simulink model "sampleModel1596_5"  (R2023a)
settings: Solver=VariableStepAuto  StartTime=0.0  StopTime=10.0  RelTol=1e-3
libraries: simulink x2, hdlsllib x2
settings Model: Creator=user1  LastModifiedBy=user1

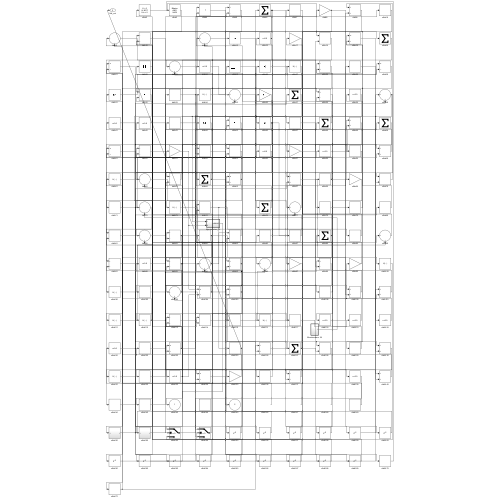
[thumbnail: Simulink's stored preview of the top-level diagram]
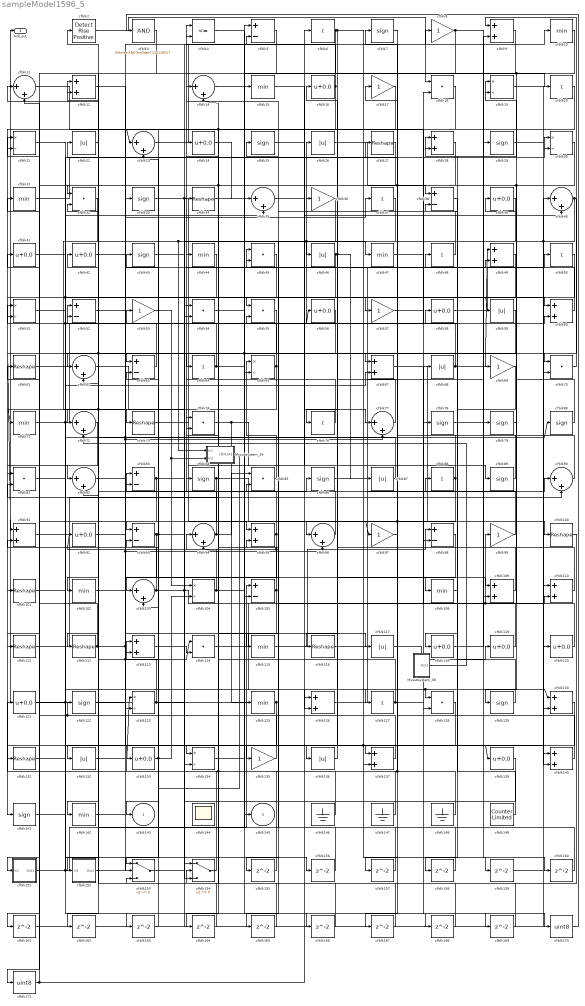
== system sampleModel1596_5 ==
  Mysubsystem_24 : Subsystem  TreatAsAtomicUnit=on  RTWFcnName=Mysubsystem_24
      settings: RTWFcnNameOpts=User specified  RTWFileNameOpts=Use function name
  Mysubsystem_38 : Subsystem  TreatAsAtomicUnit=on  RTWFcnName=Mysubsystem_38
      settings: RTWFcnNameOpts=User specified  RTWFileNameOpts=Use function name
  cfblk{10,15,31,44,47,71,102,108,115,125,142} (11 alike) : MinMax  OutDataTypeStr=uint8
  cfblk{27,34,61,73,100..101,111..112,116,131} (10 alike) : Reshape
  cfblk{11,14,23,35,40,62,72,77,82,90,94,96,103} (13 alike) : Sum  Inputs=|++  OutDataTypeStr=uint8
  cfblk{19,21,30,51,65,104,123,134} (8 alike) : Product  Inputs=*/  OutDataTypeStr=uint8  RndMeth=Zero  SaturateOnIntegerOverflow=on
  cfblk{5,38,52,63,83,93,98,105} (8 alike) : Sum  Inputs=+-  OutDataTypeStr=uint8
  cfblk{9,12,28,49,60,67,91,95,109..110,113,126,130,137,140} (15 alike) : Sum  OutDataTypeStr=uint8
  cfblk{18,32,45,54..55,70,74,81,85,114,128} (11 alike) : DotProduct  OutDataTypeStr=uint8
  cfblk{22,26,46,59,68,87,117,132,136} (9 alike) : Abs  OutDataTypeStr=uint8  SaturateOnIntegerOverflow=off
  cfblk{16,24,39,41..42,56,58,92,118..121,133,139} (14 alike) : Bias  Bias=0.0  SaturateOnIntegerOverflow=off
  cfblk{7,25,29,33,43,78..80,84,86,89,122,129,141} (14 alike) : Signum
  cfblk{6,20,37,48,50,64,76,88,127} (9 alike) : Sum  Inputs=+  OutDataTypeStr=uint8
  cfblk{8,17,36,53,57,69,97,99,135} (9 alike) : Gain  OutDataTypeStr=uint8
  cfblk144 : Scope
      settings: Floating=on
  cfblk146 : Ground
  cfblk147 : Ground
  cfblk148 : Ground
  cfblk149 : hdlsllib/Sources/Counter Limited  uplimit=7  tsamp=-1
  cfblk151 : Subsystem
      settings: LibrarySourceBlock=|
      | hdlsllib/Ports &
      | Subsystems/Subsystem
  cfblk152 : Subsystem
      settings: LibrarySourceBlock=|
      | hdlsllib/Ports &
      | Subsystems/Subsystem
  cfblk153 : Switch  OutDataTypeStr=uint8  SaturateOnIntegerOverflow=off  InputSameDT=off
  cfblk154 : Switch  OutDataTypeStr=uint8  SaturateOnIntegerOverflow=off  InputSameDT=off
  cfblk{155..169} (15 alike) : Delay  SampleTime=1
  cfblk170 : DataTypeConversion  OutDataTypeStr=uint8  SaturateOnIntegerOverflow=off  RndMeth=Floor
  cfblk171 : DataTypeConversion  OutDataTypeStr=uint8  SaturateOnIntegerOverflow=off  RndMeth=Floor
  cfblk2 : hdlsllib/Logic and Bit Operations/Detect Rise Positive  vinit=0  OutDataTypeStr=uint8
  cfblk3 : simulink/Logic and Bit Operations/Bitwise Operator  logicop=AND  UseBitMask=on  BitMask=bin2dec('11011001')  BitMaskRealWorld=Stored Integer
      settings: LibrarySourceBlock=|
      | hdlsllib/Logic and Bit
      | Operations/Bitwise
      | Operator
  cfblk4 : RelationalOperator  Operator=<=  OutDataTypeStr=boolean  InputSameDT=off
  cfblk143 : Outport  OutDataTypeStr=uint8  VectorParamsAs1DForOutWhenUnconnected=off
  cfblk145 : Outport  Port=2  OutDataTypeStr=uint8  VectorParamsAs1DForOutWhenUnconnected=off
  Hdl_out : Outport  Port=3  OutDataTypeStr=uint8
  wires:
  cfblk115/1 -> cfblk98/1
  cfblk53/1 -> cfblk104/1, Mysubsystem_24/2(In2)
  cfblk95/1 -> cfblk4/1, cfblk103/2
  cfblk65/1 -> cfblk71/1, cfblk162/1, cfblk24/1
  cfblk2/1 -> cfblk18/1
  cfblk126/1 -> cfblk48/1
  cfblk6/1 -> cfblk96/1, cfblk159/1, cfblk32/1
  cfblk148/1 -> cfblk123/1, cfblk17/1
  cfblk23/1 -> cfblk10/1
  cfblk110/1 -> cfblk52/1
  cfblk38/1 -> cfblk118/1
  cfblk45/1 -> cfblk133/1
  cfblk68/1 -> cfblk49/1, cfblk51/2
  cfblk33/1 -> cfblk139/1, cfblk137/2, cfblk95/1
  cfblk132/1 -> cfblk114/1, cfblk37/1
  cfblk137/1 -> cfblk113/1
  cfblk32/1 -> cfblk73/1
  cfblk5/1 -> cfblk142/1
  cfblk72/1 -> cfblk141/1
  cfblk74/1 -> cfblk127/1, cfblk125/1
  cfblk113/1 -> cfblk114/2
  cfblk24/1 -> cfblk35/1
  cfblk117/1 -> cfblk119/1
  cfblk76/1 -> cfblk34/1
  cfblk85/1 -> cfblk65/1
  cfblk90/1 -> cfblk22/1
  cfblk93/1 -> cfblk63/2, cfblk85/2, cfblk123/2
  cfblk135/1 -> cfblk122/1, cfblk41/1
  cfblk47/1 -> cfblk98/2
  cfblk26/1 -> cfblk38/1
  cfblk96/1 -> cfblk11/1
  cfblk88/1 -> cfblk44/1, cfblk112/1
  cfblk62/1 -> cfblk154/1
  cfblk18/1 -> cfblk93/1
  cfblk94/1 -> cfblk43/1, cfblk85/1
  cfblk151/1(Out1) -> cfblk105/1, cfblk67/2
  cfblk60/1 -> cfblk25/1
  cfblk71/1 -> cfblk26/1, cfblk140/2
  cfblk43/1 -> cfblk47/1
  cfblk83/1 -> cfblk49/2, cfblk161/1
  cfblk9/1 -> cfblk67/1
  cfblk92/1 -> cfblk8/1, cfblk77/2
  cfblk63/1 -> cfblk11/2
  cfblk127/1 -> cfblk84/1, cfblk169/1
  cfblk89/1 -> cfblk53/1
  cfblk10/1 -> cfblk28/1, cfblk167/1
  cfblk27/1 -> cfblk72/1
  cfblk77/1 -> cfblk16/1
  cfblk21/1 -> cfblk128/1, cfblk130/1, cfblk59/1
  cfblk44/1 -> cfblk153/1
  cfblk52/1 -> cfblk64/1
  cfblk73/1 -> cfblk128/2
  cfblk25/1 -> cfblk40/2
  cfblk67/1 -> cfblk100/1
  cfblk39/1 -> Mysubsystem_24/1(In1), cfblk62/2
  cfblk79/1 -> cfblk19/1
  cfblk133/1 -> cfblk83/1, cfblk104/2
  cfblk114/1 -> cfblk68/1
  cfblk3/1 -> cfblk171/1
  cfblk11/1 -> cfblk78/1
  cfblk123/1 -> cfblk12/1, cfblk60/2
  cfblk48/1 -> cfblk14/1
  cfblk149/1 -> cfblk28/2
  cfblk99/1 -> cfblk42/1
  cfblk70/1 -> cfblk9/1
  cfblk41/1 -> cfblk65/2, cfblk70/2
  cfblk128/1 -> cfblk151/1(In1)
  cfblk147/1 -> cfblk14/2, cfblk61/1
  cfblk116/1 -> cfblk90/1
  cfblk15/1 -> cfblk89/1
  cfblk87/1 -> cfblk2/1
  cfblk31/1 -> cfblk30/1
  cfblk59/1 -> cfblk82/1, cfblk91/1
  cfblk34/1 -> cfblk15/1
  cfblk146/1 -> cfblk121/1
  cfblk103/1 -> cfblk110/2, cfblk117/1, cfblk51/1
  cfblk40/1 -> cfblk54/2, cfblk130/2, cfblk70/1
  cfblk30/1 -> cfblk152/1(In1), cfblk129/1
  cfblk16/1 -> cfblk101/1, cfblk4/2
  cfblk142/1 -> cfblk33/1
  cfblk42/1 -> cfblk115/1, cfblk96/2
  cfblk129/1 -> cfblk38/2
  cfblk28/1 -> cfblk111/1, cfblk134/1, cfblk57/1
  cfblk81/1 -> cfblk35/2
  cfblk78/1 -> cfblk9/2
  cfblk80/1 -> cfblk19/2
  cfblk8/1 -> cfblk102/1, cfblk160/1
  cfblk97/1 -> cfblk137/1
  cfblk109/1 -> cfblk58/1
  cfblk112/1 -> cfblk45/1, cfblk134/2, cfblk21/2
  cfblk46/1 -> cfblk76/1, cfblk87/1, cfblk81/1
  cfblk86/1 -> cfblk29/1
  cfblk152/1(Out1) -> cfblk86/1
  cfblk136/1 -> cfblk36/1
  cfblk20/1 -> cfblk23/1, cfblk94/2
  cfblk108/1 -> cfblk88/1
  cfblk12/1 -> cfblk108/1
  cfblk64/1 -> cfblk126/2, cfblk21/1
  cfblk125/1 -> cfblk132/1, Hdl_out/1
  cfblk119/1 -> cfblk99/1, cfblk45/2
  cfblk14/1 -> cfblk20/1
  cfblk104/1 -> cfblk109/1, cfblk94/1
  cfblk91/1 -> cfblk90/2
  cfblk121/1 -> cfblk74/1, cfblk153/2
  cfblk29/1 -> cfblk140/1
  cfblk58/1 -> cfblk50/1
  cfblk141/1 -> cfblk30/2, cfblk56/1
  cfblk153/1 -> cfblk5/2
  cfblk61/1 -> cfblk18/2
  cfblk22/1 -> cfblk62/1
  cfblk82/1 -> cfblk27/1
  cfblk19/1 -> cfblk120/1
  cfblk17/1 -> cfblk116/1
  cfblk4/1 -> cfblk145/1
  cfblk55/1 -> cfblk83/2
  cfblk98/1 -> cfblk136/1
  cfblk122/1 -> cfblk80/1, cfblk55/2
  cfblk57/1 -> cfblk60/1
  cfblk140/1 -> cfblk7/1
  cfblk50/1 -> cfblk105/2
  cfblk7/1 -> cfblk97/1, cfblk157/1
  cfblk111/1 -> cfblk79/1
  cfblk105/1 -> cfblk92/1, cfblk81/2, cfblk164/1
  cfblk84/1 -> cfblk103/1, cfblk109/2
  cfblk102/1 -> cfblk135/1
  cfblk56/1 -> cfblk131/1
  cfblk100/1 -> cfblk154/2
  cfblk120/1 -> cfblk39/1
  cfblk37/1 -> cfblk46/1, cfblk55/1
  cfblk36/1 -> cfblk63/1
  cfblk118/1 -> cfblk69/1
  cfblk139/1 -> cfblk154/3
  cfblk154/1 -> cfblk31/1
  cfblk35/1 -> cfblk77/1
  cfblk49/1 -> cfblk155/1
  cfblk155/1 -> cfblk113/2
  cfblk51/1 -> cfblk156/1
  cfblk156/1 -> cfblk5/1
  cfblk157/1 -> cfblk95/2
  cfblk69/1 -> cfblk158/1
  cfblk158/1 -> cfblk12/2
  cfblk159/1 -> cfblk40/1
  cfblk160/1 -> cfblk93/2
  cfblk161/1 -> cfblk54/1
  cfblk162/1 -> cfblk110/1
  cfblk101/1 -> cfblk163/1
  cfblk163/1 -> cfblk23/2
  cfblk164/1 -> cfblk32/2
  cfblk130/1 -> cfblk165/1
  cfblk165/1 -> cfblk52/2
  cfblk134/1 -> cfblk166/1
  cfblk166/1 -> cfblk126/1
  cfblk167/1 -> cfblk153/3
  cfblk131/1 -> cfblk168/1
  cfblk168/1 -> cfblk82/2
  cfblk169/1 -> cfblk74/2
  cfblk54/1 -> cfblk170/1
  cfblk170/1 -> cfblk3/1
  cfblk171/1 -> cfblk91/2, cfblk6/1
  Mysubsystem_24/1(cfblk143) -> cfblk143/1
  Mysubsystem_38/1(Out1) -> cfblk72/2

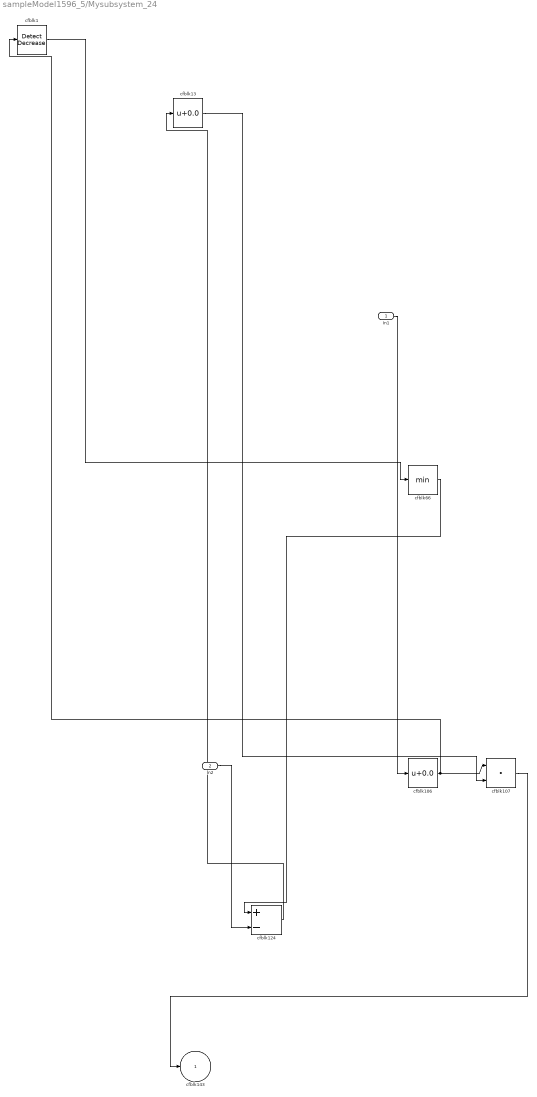
== system sampleModel1596_5/Mysubsystem_24 ==
  In1 : Inport
  In2 : Inport  Port=2
  cfblk1 : simulink/Logic and Bit Operations/Detect Decrease  vinit=0.0  OutDataTypeStr=boolean
      settings: LibrarySourceBlock=|
      | hdlsllib/Logic and Bit
      | Operations/Detect
      | Decrease
  cfblk106 : Bias  Bias=0.0  SaturateOnIntegerOverflow=off
  cfblk107 : DotProduct  OutDataTypeStr=Inherit: Inherit via internal rule
  cfblk124 : Sum  Inputs=+-
  cfblk13 : Bias  Bias=0.0  SaturateOnIntegerOverflow=off
  cfblk66 : MinMax
  cfblk143 : Outport  VectorParamsAs1DForOutWhenUnconnected=off
  wires:
  In1/1 -> cfblk106/1
  cfblk106/1 -> cfblk107/1, cfblk1/1
  cfblk66/1 -> cfblk124/1
  cfblk1/1 -> cfblk66/1
  cfblk124/1 -> cfblk13/1
  In2/1 -> cfblk124/2
  cfblk13/1 -> cfblk107/2
  cfblk107/1 -> cfblk143/1

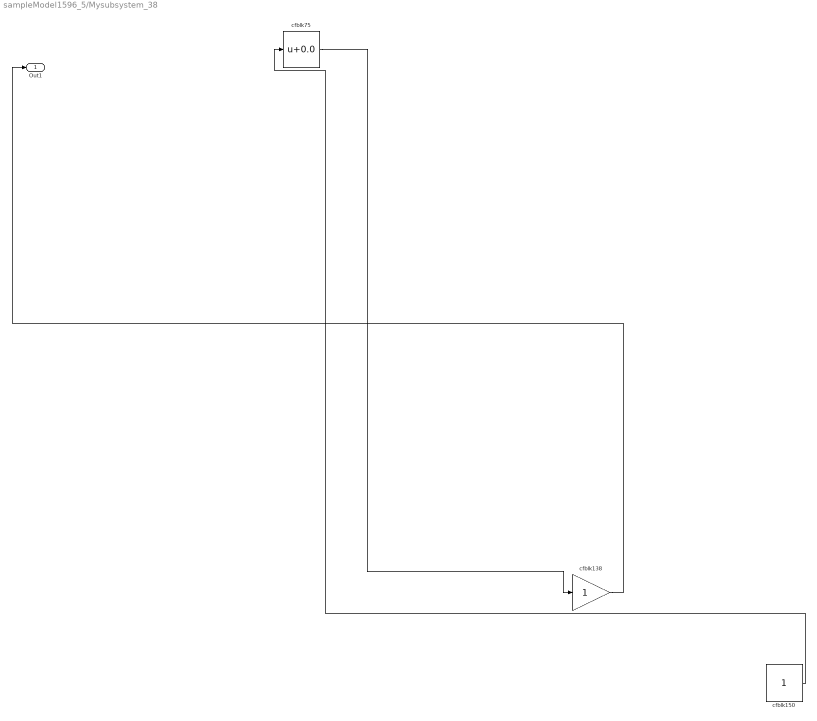
== system sampleModel1596_5/Mysubsystem_38 ==
  cfblk138 : Gain
  cfblk150 : Constant  SampleTime=-1
  cfblk75 : Bias  Bias=0.0  SaturateOnIntegerOverflow=off
  Out1 : Outport
  wires:
  cfblk138/1 -> Out1/1
  cfblk75/1 -> cfblk138/1
  cfblk150/1 -> cfblk75/1

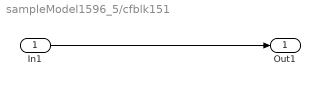
== system sampleModel1596_5/cfblk151 ==
  In1 : Inport
  Out1 : Outport
  wires:
  In1/1 -> Out1/1

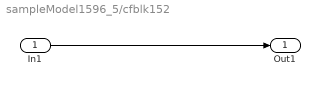
== system sampleModel1596_5/cfblk152 ==
  In1 : Inport
  Out1 : Outport
  wires:
  In1/1 -> Out1/1
